simulink model "Pendulum"  (R2019b)
settings: Solver=VariableStepAuto  StartTime=0.0  StopTime=80  RelTol=1e-3
values from neighbouring files (symbols this model uses):
  c = 0.00035    [envVariables.m]
  d = 0.023    [envVariables.m]
  g = 9.80665    [envVariables.m]
  J = 0.0090    (= 0.009)    [envVariables.m]
  L = 0.495    [envVariables.m]
  m = 0.43    [envVariables.m]
libraries: simulink x2, simulink_extras x2, fuzblock x1
settings Model: SimulationMode=rapid-accelerator  PacingRate=0.220000  Creator=victo  LastModifiedBy=victo
settings SolverCC: ZeroCrossControl=DisableAll
settings OptimizationCC: BooleanDataType=off

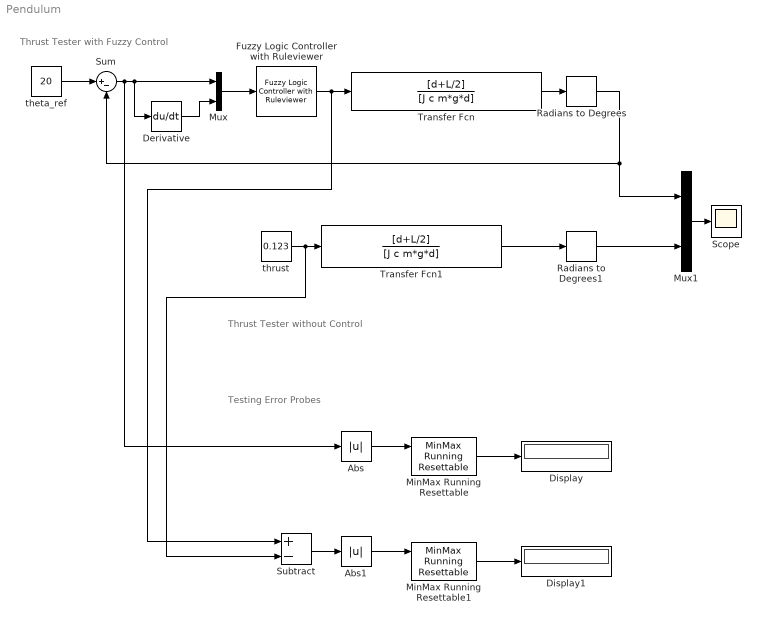
== system Pendulum ==
  note: Thrust Tester with Fuzzy Control
  note: Thrust Tester without Control
  note: Testing Error Probes
  Abs : Abs
  Abs1 : Abs
  Derivative : Derivative  CoefficientInTFapproximation=c
  Display : Display
  Display1 : Display
  Fuzzy Logic Controller with Ruleviewer : fuzblock/Fuzzy Logic  Controller  with Ruleviewer  fismatrix=output5mfFis  Ts=1
  MinMax Running Resettable : simulink/Math Operations/MinMax Running Resettable  Function=min  vinit=500000
  MinMax Running Resettable1 : simulink/Math Operations/MinMax Running Resettable  Function=min  vinit=500000
  Mux : Mux  Inputs=2
  Mux1 : Mux  Inputs=2
  Radians to Degrees : simulink_extras/Transformations/Radians to Degrees
  Radians to Degrees1 : simulink_extras/Transformations/Radians to Degrees
  Scope : Scope
  Subtract : Sum  Inputs=+-
  Sum : Sum  Inputs=|+-
  Transfer Fcn : TransferFcn  Numerator=[d+L/2]  Denominator=[J c m*g*d]
  Transfer Fcn1 : TransferFcn  Numerator=[d+L/2]  Denominator=[J c m*g*d]
  theta_ref : Constant  Value=20
  thrust : Constant  Value=0.123
  wires:
  Sum/1 -> Abs/1, Derivative/1, Mux/1
  Transfer Fcn/1 -> Radians to Degrees/1
  thrust/1 -> Subtract/2, Transfer Fcn1/1
  Transfer Fcn1/1 -> Radians to Degrees1/1
  Radians to Degrees/1 -> Sum/2, Mux1/1
  Radians to Degrees1/1 -> Mux1/2
  Mux1/1 -> Scope/1
  Derivative/1 -> Mux/2
  theta_ref/1 -> Sum/1
  Mux/1 -> Fuzzy Logic Controller with Ruleviewer/1
  Fuzzy Logic Controller with Ruleviewer/1 -> Subtract/1, Transfer Fcn/1
  Subtract/1 -> Abs1/1
  Abs/1 -> MinMax Running Resettable/1
  MinMax Running Resettable/1 -> Display/1
  Abs1/1 -> MinMax Running Resettable1/1
  MinMax Running Resettable1/1 -> Display1/1
